simulink model "DigitalModulation_PSK"  (R2023b)
settings: Solver=VariableStepAuto  StartTime=0.0  StopTime=10.0  RelTol=1e-3
settings Model: Creator=Aman Tripathi  LastModifiedBy=Spedrik Webster

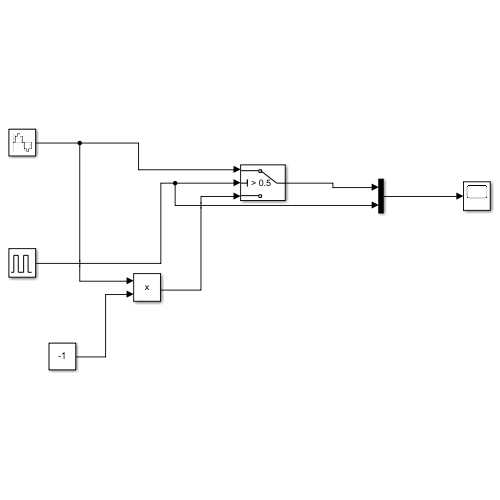
[thumbnail: Simulink's stored preview of the top-level diagram]
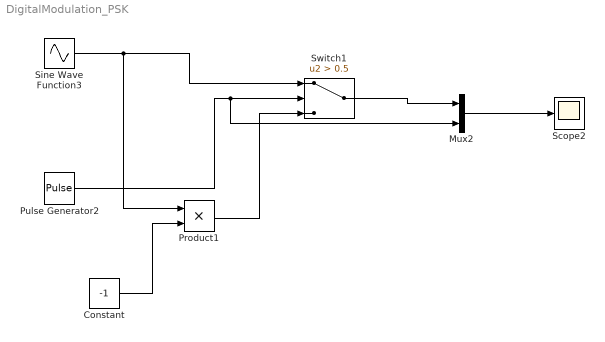
== system DigitalModulation_PSK ==
  Constant : Constant  Value=-1
  Mux2 : Mux  Inputs=2
  Product1 : Product
  Pulse Generator2 : DiscretePulseGenerator  PulseType=Time based  PulseWidth=50
  Scope2 : Scope
  Sine Wave Function3 : Sin  Frequency=10  SampleTime=1/5000
  Switch1 : Switch  Criteria=u2 > Threshold  Threshold=0.5  SaturateOnIntegerOverflow=off  InputSameDT=off
  wires:
  Sine Wave Function3/1 -> Product1/1, Switch1/1
  Product1/1 -> Switch1/3
  Pulse Generator2/1 -> Mux2/2, Switch1/2
  Constant/1 -> Product1/2
  Mux2/1 -> Scope2/1
  Switch1/1 -> Mux2/1
